simulink model "Lidar_System_FullState_Sep26Triangle"  (Simulink 7.3)
settings: Solver=FixedStepDiscrete  StartTime=0.0  StopTime=inf  FixedStep=0.1  MaxStep=0.2  RelTol=1e-3
undefined symbols (not defined in the file): strel
libraries: dspmtrx3 x9, simulink x7, vipstatistics x3, vipmorphops x3, dspstat3 x3, dspindex x1
(part 2 of 2)

== matlab function Enabled Subsystem1/Embedded MATLAB Function ==
  data: potVal input double; yn output double
function yn = check_pot_val(potVal)
%#eml

% Pot value may initially be zero.
% Check for this and output a 1 or zero to 
% control whether the rest of model runs
if (potVal == 0)
    yn = 0;
else
    yn = 1;
end

== matlab function Enabled Subsystem1/Stepper Speed and Postion Calculation ==
  data: UpAngle input double; Speed output double; DownAngle input double; Upos output double; Dpos output double; ScanNum output double; Scans input double
function [Speed,Upos,Dpos,ScanNum] = stepper_calc(UpAngle,DownAngle,Scans)
% Last Edited by Anderson Lebbad on July 7, 2014
% edits were made to account for new calibration on gimbal

% This function inputs desired positive and negative scan angles
% and desired number of scans and outputs results positions for
% the stepper and the required speed of the stepper motor to properly
% move so the desired number of scans is obtained over the course of
% the motion of the stepper


% Pass scan Number
ScanNum = Scans;
% Number of steps for 180 degree flip
stepRes = 7326;
% Parameter to account for slack in the gears with respect to steps
stepGive = 57;

% Transformation of angle to stepper position obtained from stepper calibration
% Output must be an integer
% 57 is added or subtracted due to wobble of gimbal system
Upos = -round(UpAngle*stepRes/180)-stepGive;
Dpos = -round(DownAngle*stepRes/180)+stepGive;

% Speed Calculation
% Output must be an interger
Speed = round(abs(UpAngle-DownAngle) * (2145-((65-Scans)/6))/90 * 65/Scans);

== matlab function Enabled Subsystem1/Perception/Color Analysis/Template Matching (Docking)/Docking2/Recognition/Embedded MATLAB Function ==
  data: targetTemp input double; bbox_out output double; cruciform input double; circle input double; triangle input double; whitePixCount input double; threshold input double; V_mask input double; bbox_in input double; returnRatioDiff output double
function [bbox_out,returnRatioDiff] = recognition(targetTemp,cruciform,circle,triangle,...
    whitePixCount,threshold,V_mask,bbox_in)

% Written by Edward Zhu on 5/14/14

% Inputs
% tempID:       Number corresponding to one of the templates (cruciform: 1,
%               circle: 2, triangle: 3)
% cruciform:    19*19 template of cruciform
% circle:       19*19 template of circle
% triangle:     19*19 template of triangle
% whitePixCount:Number of white pixels in each of the templates
% V_mask:       V channel binary mask
% bbox_in:      Bounding boxes as found by blob analysis
% label:        Label matrix as found by blob analysis

% Outputs
% bbox_out:     Bounding box of matched symbol
% symFound:     Status of matching (found: 1, not found: 0)

% Define frame and template size
templates = zeros(19,19,3);
templates(:,:,1) = cruciform;
templates(:,:,2) = circle;
templates(:,:,3) = triangle;
templates = 2*(templates-0.5);

tempRows = size(templates,1);
tempCols = size(templates,2);
numBBox = size(bbox_in,1);

% Initialize scaled image and output bbox matrices
V_scaled = zeros(tempRows,tempCols);
bbox_out = uint32(zeros(numBBox,4));

returnRatioDiff = ones(numBBox,1);

for i = 1:numBBox
       
    if (min(bbox_in(i,:)) > 0 && (bbox_in(i,1)+bbox_in(i,3)) < 640  && (bbox_in(i,2) + bbox_in(i,4) < 480))
        similarity = 0;
        rowScaleStep = floor(bbox_in(i,4) / tempRows);
        colScaleStep = floor(bbox_in(i,3) / tempCols);
        
        captureRow = bbox_in(i,2);
        for row = 1:tempRows
            captureCol = bbox_in(i,1);
            if (captureCol > 640)
                captureCol = uint32(640);
            end
            if (captureRow > 480)
                captureRow = uint32(480);
            end
            for col = 1:tempCols
                V_scaled(row,col) = V_mask(captureRow,captureCol);
                similarity = similarity + templates(row,col,targetTemp) * (V_mask(captureRow,captureCol)*(-1) + 1);
                captureCol = captureCol + colScaleStep;
            end
            captureRow = captureRow + rowScaleStep;
        end
        
        ratioDiff = abs(1 - single(similarity) / single(whitePixCount(targetTemp)));
        
        % Output valid bounding box
        if ratioDiff < threshold
            bbox_out(i,:) = bbox_in(i,:);
            returnRatioDiff(i) = ratioDiff;
        end
    end
end
